simulink model "lti_aumentado2"  (R2023b)
settings: Solver=VariableStepAuto  StartTime=0.0  StopTime=10.0  RelTol=1e-3
values from neighbouring files (symbols this model uses):
  b_eq = b_eq_max    (= 2.40277777778e-05)    [analisis_estabilidad.m]    (also in parametros.m = 2.19444444444e-05; parametros_sim.m = 2.19444444444e-05)
  C_ts = 0.818    [analisis_estabilidad.m]    (also in parametros.m; parametros_sim.m)
  J_eq = J_eq_max    (= 4.58263888889e-05)    [analisis_estabilidad.m]    (also in parametros.m = 1.97847222222e-05; parametros_sim.m = 1.97847222222e-05)
  L_d = 6.6    [analisis_estabilidad.m]    (also in parametros.m = 0.0066; parametros_sim.m; polosyceros.m = L_d^3)
  L_ls = 0.8    [analisis_estabilidad.m]    (also in parametros.m = 0.0008; parametros_sim.m)
  L_q = 5.8    [analisis_estabilidad.m]    (also in parametros.m = 0.0058; parametros_sim.m; polosyceros.m = L_q^3)
  lambda_m = 0.016    [analisis_estabilidad.m]    (also in parametros.m; parametros_sim.m)
  P_p = 3    [analisis_estabilidad.m]    (also in parametros.m; parametros_sim.m)
  r = 120    [analisis_estabilidad.m]    (also in parametros.m; parametros_sim.m)
  R_s = R_s_max    (= 1.39791)    [analisis_estabilidad.m]    (also in frec_nat_y_amort.m = R_s_ref * (1 + alpha_Cu * (T - T_s_ref)); parametros.m = 1.02)
  R_ts_amb = 146.7    [analisis_estabilidad.m]    (also in parametros.m; parametros_sim.m)
settings Model: Creator=Marti  LastModifiedBy=Marti

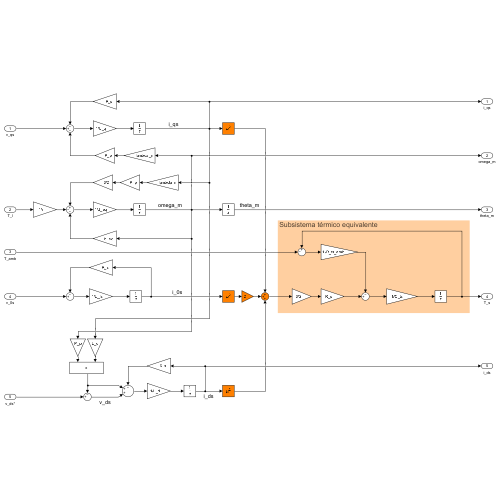
[thumbnail: Simulink's stored preview of the top-level diagram]
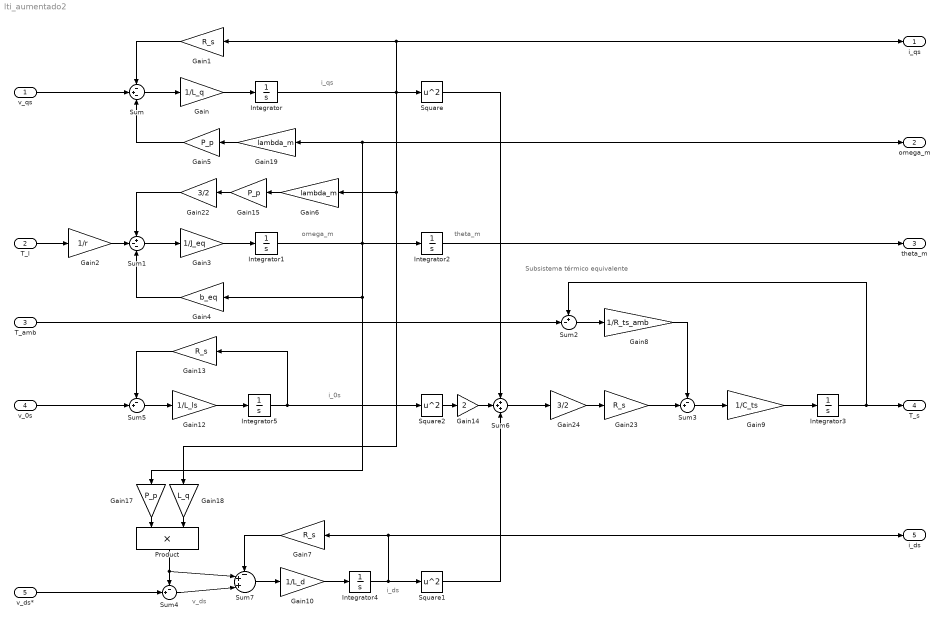
== system lti_aumentado2 ==
  note: i_qs
  note: omega_m
  note: i_0s
  note: Subsistema térmico equivalente
  note: theta_m
  note: v_ds
  note: i_ds
  v_qs : Inport
  T_l : Inport  Port=2
  T_amb : Inport  Port=3
  v_0s : Inport  Port=4
  v_ds* : Inport  Port=5
  Gain : Gain  Gain=1/L_q
  Gain{1,7,13,23} (4 alike) : Gain  Gain=R_s
  Gain10 : Gain  Gain=1/L_d
  Gain12 : Gain  Gain=1/L_ls
  Gain14 : Gain  Gain=2
  Gain15 : Gain  Gain=P_p
  Gain17 : Gain  Gain=P_p
  Gain18 : Gain  Gain=L_q
  Gain19 : Gain  Gain=lambda_m
  Gain2 : Gain  Gain=1/r
  Gain22 : Gain  Gain=3/2
  Gain24 : Gain  Gain=3/2
  Gain3 : Gain  Gain=1/J_eq
  Gain4 : Gain  Gain=b_eq
  Gain5 : Gain  Gain=P_p
  Gain6 : Gain  Gain=lambda_m
  Gain8 : Gain  Gain=1/R_ts_amb
  Gain9 : Gain  Gain=1/C_ts
  Integrator{,1..5} (6 alike) : Integrator
  Product : Product
  Square : Math  Operator=square
  Square1 : Math  Operator=square
  Square2 : Math  Operator=square
  Sum : Sum  Inputs=-+-
  Sum1 : Sum  Inputs=+--
  Sum2 : Sum  Inputs=+-|
  Sum3 : Sum  Inputs=-+|
  Sum4 : Sum  Inputs=-+|
  Sum5 : Sum  Inputs=-+|
  Sum6 : Sum  Inputs=+++
  Sum7 : Sum  Inputs=-++|
  i_qs : Outport
  omega_m : Outport  Port=2
  theta_m : Outport  Port=3
  T_s : Outport  Port=4
  i_ds : Outport  Port=5
  wires:
  Gain13/1 -> Sum5/1
  Sum2/1 -> Gain8/1
  Integrator1/1 -> Gain19/1, omega_m/1, Integrator2/1, Gain4/1, Gain17/1
  Gain19/1 -> Gain5/1
  Gain2/1 -> Sum1/2
  Gain4/1 -> Sum1/3
  Gain5/1 -> Sum/3
  v_qs/1 -> Sum/2
  Integrator/1 -> Gain1/1, i_qs/1, Square/1, Gain6/1, Gain18/1
  Square/1 -> Sum6/1
  Gain1/1 -> Sum/1
  Sum/1 -> Gain/1
  T_amb/1 -> Sum2/2
  Sum5/1 -> Gain12/1
  Gain8/1 -> Sum3/1
  Gain9/1 -> Integrator3/1
  Sum3/1 -> Gain9/1
  Square2/1 -> Gain14/1
  Integrator3/1 -> Sum2/1, T_s/1
  Gain3/1 -> Integrator1/1
  Gain12/1 -> Integrator5/1
  Integrator5/1 -> Square2/1, Gain13/1
  T_l/1 -> Gain2/1
  Sum1/1 -> Gain3/1
  Gain/1 -> Integrator/1
  v_0s/1 -> Sum5/2
  Gain22/1 -> Sum1/1
  Gain15/1 -> Gain22/1
  Gain6/1 -> Gain15/1
  Integrator2/1 -> theta_m/1
  Gain14/1 -> Sum6/2
  Gain24/1 -> Gain23/1
  Gain23/1 -> Sum3/2
  Sum6/1 -> Gain24/1
  v_ds*/1 -> Sum4/2
  Gain18/1 -> Product/2
  Gain17/1 -> Product/1
  Product/1 -> Sum7/2, Sum4/1
  Sum4/1 -> Sum7/3
  Sum7/1 -> Gain10/1
  Gain10/1 -> Integrator4/1
  Integrator4/1 -> Square1/1, i_ds/1, Gain7/1
  Gain7/1 -> Sum7/1
  Square1/1 -> Sum6/3
